simulink model "c_prog_3057"  (R2018b)
settings: Solver=VariableStepAuto  StartTime=0.0  StopTime=10.0  RelTol=1e-3
settings Model: Creator=student  LastModifiedBy=student

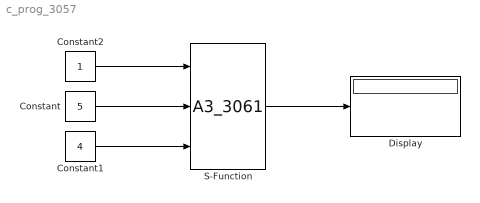
== system c_prog_3057 ==
  Constant : Constant  Value=5
  Constant1 : Constant  Value=4
  Constant2 : Constant
  Display : Display
  S-Function : S-Function  FunctionName=A3_3061  SFunctionDeploymentMode=off  EnableBusSupport=off
  wires:
  Constant2/1 -> S-Function/1
  Constant/1 -> S-Function/2
  Constant1/1 -> S-Function/3
  S-Function/1 -> Display/1
